simulink model "Dynamic_vib_abs"  (R2020a)
settings: Solver=VariableStepAuto  StartTime=0.0  StopTime=10.0  RelTol=1e-3
values from neighbouring files (symbols this model uses):
  b = 50    [command window.mat]
  k1 = 50    [command window.mat]
  k12 = -0.0202546256444    [command window.mat]
  m1 = 0.01    [command window.mat]
  m2 = -4937.14382856    [command window.mat]
settings Model: Creator=kolep  LastModifiedBy=kolep

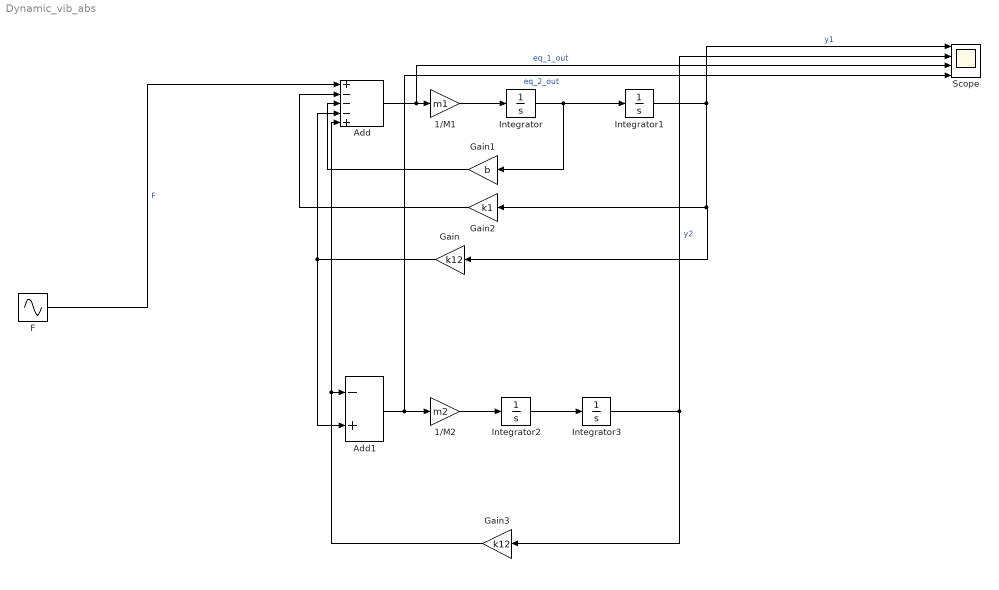
== system Dynamic_vib_abs ==
  1/M1 : Gain  Gain=m1
  1/M2 : Gain  Gain=m2
  Add : Sum  Inputs=+---+
  Add1 : Sum  Inputs=-+
  F : Sin  Amplitude=2  Frequency=10  SampleTime=0
  Gain : Gain  Gain=k12
  Gain1 : Gain  Gain=b
  Gain2 : Gain  Gain=k1
  Gain3 : Gain  Gain=k12
  Integrator{,1..3} (4 alike) : Integrator
  Scope : Scope  NumInputPorts=4
  wires:
  Gain/1 -> Add1/2, Add/4
  1/M2/1 -> Integrator2/1
  Gain2/1 -> Add/2
  Gain3/1 -> Add/5, Add1/1
  Gain1/1 -> Add/3
  Integrator1/1 -> Scope/1, Gain2/1, Gain/1  "y1"
  Integrator3/1 -> Scope/2, Gain3/1  "y2"
  Add/1 -> Scope/3, 1/M1/1  "eq_1_out"
  Integrator2/1 -> Integrator3/1
  Integrator/1 -> Integrator1/1, Gain1/1
  Add1/1 -> Scope/4, 1/M2/1  "eq_2_out"
  1/M1/1 -> Integrator/1
  F/1 -> Add/1  "F"
